simulink model "twoFingerTCTest"  (R2015b)
settings: Solver=ode45  StartTime=0.0  StopTime=2  RelTol=1e-3
libraries: RCTblocks x3
(part 2 of 2)

== matlab function twoFingerTCTest/Index/IndexFinger/MATLAB Function ==
  data: FcSense input; fcD output; theta input
function fcD = forceConversion(FcSense,theta)
    % Transform forces:
    % Contact force
    fcTN = rotMat(theta(1,1)+theta(2,1))'*-FcSense;
    fcD = fcTN(2,1);
end
        function rot = rotMat(theta)
            % 2D Z-Rotation matrix on theta.
            % @param theta the angle
            % @return rot the rotation matrix as a 2x2 matrix.
            rot = [cos(theta) -sin(theta);
                   sin(theta) cos(theta)];
        end

== matlab function twoFingerTCTest/Subsystem/MATLAB Function8 ==
  data: r input; pos output
function pos = fcn(r)
%#codegen
    pos=[0;r];
end
